simulink model "pendu_partial_feed_colocated"  (R2018a)
settings: Solver=VariableStepAuto  StartTime=0.0  StopTime=5  RelTol=1e-3
undefined symbols (not defined in the file or in its folder): K, par, q0
settings Model: Creator=Pimentel  LastModifiedBy=Pimentel

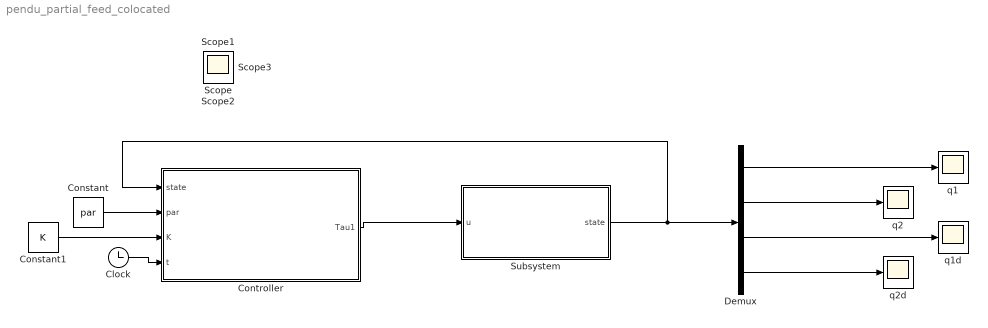
== system pendu_partial_feed_colocated ==
  Clock : Clock
  Constant : Constant  Value=par
  Constant1 : Constant  Value=K
  Controller : MATLAB Function  TreatAsAtomicUnit=on
  Demux : Demux
  Subsystem : Subsystem
  "q1 " : Scope
  q1d : Scope
  q2 : Scope
  q2d : Scope
  Scope{,1..3} (4 alike) : Scope
  wires:
  Subsystem/1(state) -> Controller/1(state), Demux/1
  Controller/1(Tau1) -> Subsystem/1("u ")
  Constant/1 -> Controller/2(par)
  Clock/1 -> Controller/4(t)
  Demux/4 -> q2d/1
  Demux/1 -> "q1 "/1
  Demux/3 -> q1d/1
  Demux/2 -> q2/1
  Constant1/1 -> Controller/3(K)

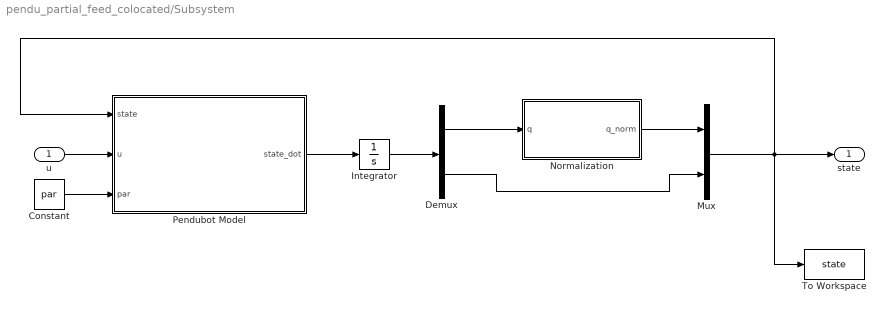
== system pendu_partial_feed_colocated/Subsystem ==
  "u " : Inport
  Constant : Constant  Value=par
  Demux : Demux  Outputs=[2 2]
  Integrator : Integrator  InitialCondition=q0
  Mux : Mux  Inputs=[2 2]
  "Normalization " : MATLAB Function  TreatAsAtomicUnit=on
  Pendubot Model : MATLAB Function  TreatAsAtomicUnit=on
  To Workspace : ToWorkspace  VariableName=state  SaveFormat=Structure With Time  SampleTime=-1
  state : Outport
  wires:
  Constant/1 -> Pendubot Model/3(par)
  "u "/1 -> Pendubot Model/2(u)
  Pendubot Model/1(state_dot) -> Integrator/1
  Integrator/1 -> Demux/1
  "Normalization "/1(q_norm) -> Mux/1
  Demux/1 -> "Normalization "/1(q)
  Mux/1 -> To Workspace/1, Pendubot Model/1(state), state/1
  Demux/2 -> Mux/2

== matlab function pendu_partial_feed_colocated/Controller ==
  data: state input; Tau1 output; par input; K input; t input
function Tau1 = controller(state,par,K,t)

% Parameters of Acrobot

m1 = par(1);
m2 = par(2);
l1 = par(3);
l2 = par(4);
lc1 = par(5);
lc2 = par(6);
I1 = par(7);
I2 = par(8);
g = par(9);

% State 

q1 = state(1);
q2 = state(2);
qd1 = state(3);
qd2 = state(4);

% Dynamic Equations elements

d11 = m1*lc1^2 + m2*(l1^2 + lc2^2 + 2*l1*lc2*cos(q2)) + I1 + I2;
d12 = m2*(lc2^2 + l1*lc2*cos(q2)) + I2;
d21 = d12;
d22 = m2*lc2^2 + I2;

h1 = -m2*l1*lc2*sin(q2)*qd2^2 - 2*m2*l1*lc2*sin(q2)*qd2*qd1;
h2 = m2*l1*lc2*sin(q2)*qd1^2;

phi1 = (m1*lc1 + m2*l1)*g*cos(q1) + m2*lc2*g*cos(q1+q2);
phi2 = m2*lc2*g*cos(q1+q2);

n1 = h1+phi1;
n2 = h2+phi2;

% Desired Final Conditions: Up-Up Position

q1_d = pi/2;
qd1_d = 0;
q2_d = 0;
qd2_d = 0;

% Controller set of Gains

kp = 28;
kd = 5;

% Partial-Feedback Linearizing Controller, Colocated Case (y = q1)

alpha = d11 - d12*d21/d22;
beta = n1 - d12/d22*n2;

v1 = kp*(q1_d - q1) + kd*(qd1_d - qd1); % Outer-Loop Control Term

if t>=1.5
    Tau1 = -K'*[q1-q1_d; q2; qd1; qd2]; % LQR Ballancing controller
else
    Tau1 = alpha*v1 + beta;
end

== matlab function pendu_partial_feed_colocated/Subsystem/Pendubot Model ==
  data: state input; u input; state_dot output; par input
function state_dot = pendubot(state, u, par)

% Parameters of Acrobot

m1 = par(1);
m2 = par(2);
l1 = par(3);
l2 = par(4);
lc1 = par(5);
lc2 = par(6);
I1 = par(7);
I2 = par(8);
g = par(9);

% State 

q1 = state(1);
q2 = state(2);
qd1 = state(3);
qd2 = state(4);

% Inertia Matrix 

d11 = m1*lc1^2 + m2*(l1^2 + lc2^2+2*l1*lc2*cos(q2)) + I1 + I2;
d12 = m2*(lc2^2 + l1*lc2*cos(q2)) + I2;
d21 = d12;
d22 = m2*lc2^2 + I2;

D = [d11, d12; d21, d22];

% Coriolis and Centrifugal terms

h1 = -m2*l1*lc2*sin(q2)*qd2^2 - 2*m2*l1*lc2*sin(q2)*qd2*qd1;
h2 = m2*l1*lc2*sin(q2)*qd1^2;

H = [h1; h2];

% Gravity terms

phi1 = (m1*lc1 + m2*l1)*g*cos(q1) + m2*lc2*g*cos(q1+q2);
phi2 = m2*lc2*g*cos(q1+q2);

Phi = [phi1; phi2];

% Invert Dynamic Euler-Lagrange equation: D(q).qdd + H(q,qd) + Phi(q) = Tau, 
% to obtain system dynamics

Tau = [u; 0];

qdd = inv(D)*(Tau - H - Phi);

state_dot = [qd1, qd2, qdd(1), qdd(2)]';

== matlab function pendu_partial_feed_colocated/Subsystem/Normalization  ==
  data: q input; q_norm output
function q_norm = norm(q)

q1 = q(1);
q2 = q(2);

% Normalization of angles between 0 and 2pi, while maintaining the sign

if q1 >= 0
    q1 = mod(q1, 2*pi);    
else
    q1 = mod(q1, -2*pi);
end

if q2 >= 0
    q2 = mod(q2, 2*pi);
else
    q2 = mod(q2, -2*pi);
end

q_norm = [q1, q2];
